simulink model "Loops7"  (Simulink 8.7)
settings: Solver=ode45  StartTime=0.0  StopTime=10.0  RelTol=1e-3
settings Model: Creator=scaife  LastModifiedBy=bourbouh  ExtModeAutoUpdateStatusClock=off
settings DataIOCC: SignalLoggingSaveFormat=ModelDataLogs  SignalLoggingName=sigsOut
settings OptimizationCC: InitFltsAndDblsToZero=on
settings DebuggingCC: SaveWithParameterizedLinksMsg=none  SignalResolutionControl=TryResolveAllWithWarning  MultiTaskDSMMsg=warning  MultiTaskCondExecSysMsg=none
settings HardwareCC: TargetUnknown=on
settings SFSimCC: SimParseCustomCode=off
settings GRTTargetCC: TargetFcnLib=ansi_tfl_tmw.mat  ModelReferenceCompliant=off  ParMdlRefBuildCompliant=off  CompOptLevelCompliant=off  ConcurrentExecutionCompliant=off  GeneratePreprocessorConditionals=Use local settings  CombineOutputUpdateFcns=off  MatFileLogging=off  MATLABClassNameForMDSCustomization=Simulink.SoftwareTarget.TargetSpecificTriggerConfigurationBase  GRTInterface=on

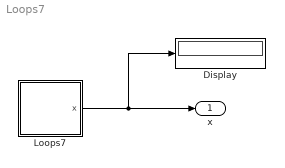
== system Loops7 ==
  Display : Display
  Loops7 : Stateflow chart  TreatAsAtomicUnit=on
  x : Outport
  wires:
  Loops7/1(x) -> x/1, Display/1

== stateflow chart Loops7 ==
  state A
  state B
  (default) -> A
  A -> (junction 6) : {x=0}
  (junction 6) -> (junction 6) [order 1] : [x<3]{x++}
  (junction 6) -> (junction 7) [order 2]
  (junction 8) -> (junction 7) [order 1] : [x<6]
  (junction 7) -> (junction 8) : {x++}
  (junction 8) -> B [order 2]
  data: x output int32
